simulink model "CellModel"  (R2019b)
settings: Solver=VariableStepAuto  StartTime=0.0  StopTime=2000  RelTol=1e-3
settings Model: Creator=jorge  LastModifiedBy=jorge

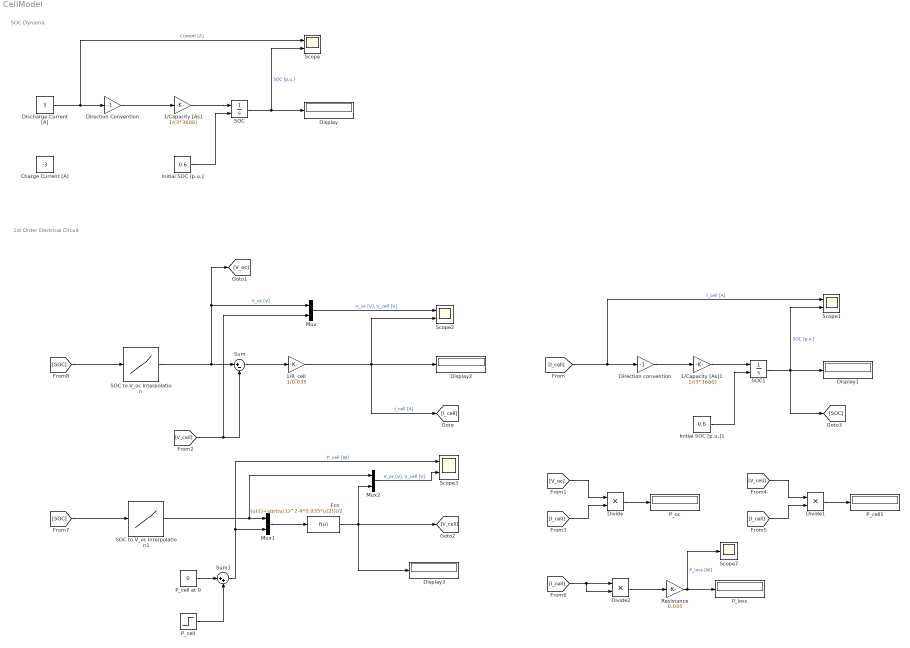
== system CellModel ==
  note: 1st Order Electrical Circuit
  note: SOC Dynamic
  1/Capacity [As] : Gain  Gain=1/(3*3600)
  1/Capacity [As]1 : Gain  Gain=1/(3*3600)
  1/R_cell : Gain  Gain=1/0.035
  Charge Current [A] : Constant  Value=-3
  Direction Convention : Gain  Gain=-1
  Direction convention : Gain  Gain=-1
  Discharge Current [A] : Constant  Value=3
  Display{,1..3} (4 alike) : Display
  Divide : Product  Inputs=**
  Divide1 : Product  Inputs=**
  Divide2 : Product  Inputs=**
  Fcn : Fcn  Expr=(u(1)+sqrt(u(1)^2-4*0.035*u(2)))/2
  Initial SOC [p.u.] : Constant  Value=0.6
  Initial SOC [p.u.]1 : Constant  Value=0.6
  Mux : Mux  Inputs=2
  Mux1 : Mux  Inputs=2
  Mux2 : Mux  Inputs=2
  P_cell : Step  After=10.8  SampleTime=0
  P_cell at 0 : Constant  Value=0
  P_cell1 : Display
  P_loss : Display
  P_oc : Display
  Resistance : Gain  Gain=0.035
  SOC : Integrator  InitialConditionSource=external  InitialCondition=0.5
  SOC to V_oc Interpolation : Lookup_n-D  NumberOfTableDimensions=1  BreakpointsForDimension1=[0,0.1,0.2,0.3,0.4,0.5,0.6,0.7,0.8,0.9,1]  UseOneInputPortForAllInputData=on  Table=[2.85,3.19,3.39,3.52,3.65,3.73,3.82,3.92,4.01,4.07,4.19]  InternalRulePriority=Speed  RndMeth=Simplest  InputSameDT=on
  SOC to V_oc Interpolation1 : Lookup_n-D  NumberOfTableDimensions=1  BreakpointsForDimension1=[0,0.1,0.2,0.3,0.4,0.5,0.6,0.7,0.8,0.9,1]  UseOneInputPortForAllInputData=on  Table=[2.85,3.19,3.39,3.52,3.65,3.73,3.82,3.92,4.01,4.07,4.19]  InternalRulePriority=Speed  RndMeth=Simplest  InputSameDT=on
  SOC1 : Integrator  InitialConditionSource=external  InitialCondition=0.5
  Scope{,1..3} (4 alike) : Scope  NumInputPorts=2
  Scope7 : Scope
  Sum : Sum  Inputs=|+-
  Sum1 : Sum  Inputs=|++
  wires:
  1/Capacity [As]/1 -> SOC/1
  SOC/1 -> Scope/2, Display/1  "SOC [p.u.]"
  Direction Convention/1 -> 1/Capacity [As]/1
  Initial SOC [p.u.]/1 -> SOC/2
  Discharge Current [A]/1 -> Scope/1, Direction Convention/1  "Current [A]"
  [I_cell] -> Scope1/1, Direction convention/1  "I_cell [A]"
  SOC1/1 -> [SOC], Scope1/2, Display1/1  "SOC [p.u.]"
  Initial SOC [p.u.]1/1 -> SOC1/2
  Direction convention/1 -> 1/Capacity [As]1/1
  1/Capacity [As]1/1 -> SOC1/1
  SOC to V_oc Interpolation/1 -> [V_oc], Mux/1, Sum/1  "V_oc [V]"
  Sum/1 -> 1/R_cell/1
  1/R_cell/1 -> Scope2/2, Display2/1, [I_cell]  "I_cell [A]"
  Mux/1 -> Scope2/1  "V_oc [V], V_cell [V]"
  [V_cell] -> Mux/2, Sum/2
  SOC to V_oc Interpolation1/1 -> Mux1/1, Mux2/1
  P_cell at 0/1 -> Sum1/1
  P_cell/1 -> Sum1/2
  Sum1/1 -> Mux1/2, Scope3/1  "P_cell [W]"
  Mux1/1 -> Fcn/1
  [V_oc] -> Divide/1
  [I_cell] -> Divide/2
  Divide/1 -> P_oc/1
  Divide1/1 -> P_cell1/1
  [V_cell] -> Divide1/1
  [I_cell] -> Divide1/2
  Fcn/1 -> Display3/1, Mux2/2, [V_cell]
  Mux2/1 -> Scope3/2  "V_oc [V], V_cell [V]"
  [I_cell] -> Divide2/2, Divide2/1
  Divide2/1 -> Resistance/1
  Resistance/1 -> P_loss/1, Scope7/1  "P_loss [W]"
  [SOC] -> SOC to V_oc Interpolation/1
  [SOC] -> SOC to V_oc Interpolation1/1
